simulink model "gm_BPSK_Modulator_Demodulator"  (R2022a)
settings: Solver=FixedStepDiscrete  StartTime=0.0  StopTime=0.1  FixedStep=2e-8  RelTol=1e-3
libraries: commdigbbndpm3 x2
settings Model: Creator=okoko  LastModifiedBy=okoko
settings OptimizationCC: BlockReduction=off  ConditionallyExecuteInputs=off  DefaultParameterBehavior=Inlined  InheritOutputTypeSmallerThanSingle=on
settings DebuggingCC: AlgebraicLoopMsg=error  InheritedTsInSrcMsg=none  SingleTaskRateTransMsg=error
settings HardwareCC: ProdBitPerPointer=32  ProdBitPerSizeT=32  ProdBitPerPtrDiffT=32  ProdLargestAtomicFloat=None  ProdIntDivRoundTo=Undefined  ProdEndianess=Unspecified  ProdWordSize=32  ProdHWDeviceType=ASIC/FPGA->ASIC/FPGA  TargetBitPerPointer=64  TargetBitPerSizeT=64  TargetBitPerPtrDiffT=64  TargetLongLongMode=on  TargetIntDivRoundTo=Zero  TargetEndianess=LittleEndian  TargetWordSize=64  TargetHWDeviceType=Custom Processor->MATLAB Host Computer  ProdEqTarget=off

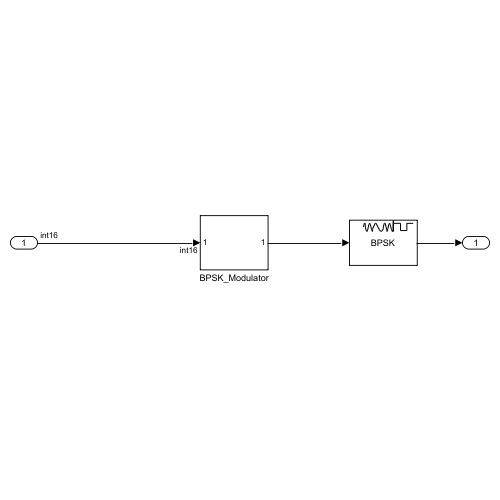
[thumbnail: Simulink's stored preview of the top-level diagram]
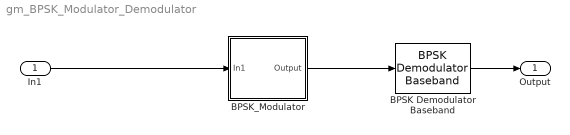
== system gm_BPSK_Modulator_Demodulator ==
  In1 : Inport  OutMin=-32768  OutMax=32767  OutDataTypeStr=int16  PortDimensions=1  SampleTime=2e-08
  BPSK Demodulator Baseband : commdigbbndpm3/BPSK Demodulator Baseband  DecType=Hard decision  VarSource=Dialog  Variance=1  Ph=0  outDtype=int16  derotateFactorWordLen=16  derotateFactorDataTypeStr=Inherit: Same word length as input  derotateFactorLastDataTypeStr=Inherit: Same word length as input
  BPSK_Modulator : Subsystem
  Output : Outport  SampleTime=2e-08
  wires:
  In1/1 -> BPSK_Modulator/1(In1)
  BPSK Demodulator Baseband/1 -> Output/1
  BPSK_Modulator/1(Output) -> BPSK Demodulator Baseband/1

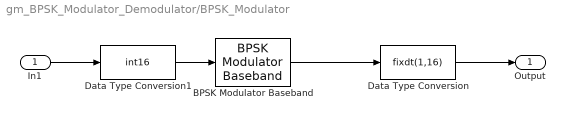
== system gm_BPSK_Modulator_Demodulator/BPSK_Modulator ==
  In1 : Inport  OutMin=-32768  OutMax=32767  OutDataTypeStr=int16  PortDimensions=1  SampleTime=2e-08
  BPSK Modulator Baseband : commdigbbndpm3/BPSK Modulator Baseband  Ph=0  outDtype=Fixed-point  outWordLen=16  outUDDataType=sfix(16)  outFracLenMode=Best precision  outFracLen=0  outDataTypeStr=fixdt(1,16)  outLastDataTypeStr=fixdt(1,16)
  Data Type Conversion : DataTypeConversion  OutMin=-32768  OutMax=32767  OutDataTypeStr=fixdt(1,16)  SaturateOnIntegerOverflow=off  RndMeth=Floor
  Data Type Conversion1 : DataTypeConversion  OutMin=-32768  OutMax=32767  OutDataTypeStr=int16  RndMeth=Nearest  SaturateOnIntegerOverflow=off
  Output : Outport  SampleTime=2e-08
  wires:
  In1/1 -> Data Type Conversion1/1
  BPSK Modulator Baseband/1 -> Data Type Conversion/1
  Data Type Conversion/1 -> Output/1
  Data Type Conversion1/1 -> BPSK Modulator Baseband/1
